simulink model "Group_11_Final_Project_model_ARO4090Rev4 (1)"  (R2023b)
settings: Solver=ode23tb  StartTime=0.0  StopTime=5676.8  FixedStep=0.002  RelTol=1e-3  EnableMultiTasking=on
undefined symbols (not defined in the file): IAU
libraries: simulink_extras x7, slpidlib x3, aerolibtransform2 x2, simulink x2
settings Model: ExtModeTrigDuration=10000  Creator=jtmil  LastModifiedBy=19095
settings SolverCC: AlgebraicLoopSolver=TrustRegion  PositivePriorityOrder=on
settings DataIOCC: ReturnWorkspaceOutputs=off
settings OptimizationCC: LifeSpan=inf
settings DebuggingCC: UnconnectedInputMsg=warning  UnconnectedOutputMsg=warning  UnconnectedLineMsg=warning  ArithmeticOperatorsInVariantConditions=warning
settings ModelReferenceCC: EnableRefExpFcnMdlSchedulingChecks=on
settings SFSimCC: SimUseLocalCustomCode=off  CustomCodeUndefinedFunction=UseInterfaceOnly
settings RTWCC: Description=QUARC Win64 Target  SystemTargetFile=quarc_win64.tlc  TemplateMakefile=quarc_default_tmf  RTWUseLocalCustomCode=off
settings CodeAppCC: StateflowObjectComments=on
settings STFCustomTargetCC: TargetPreCompLibLocation=C:\PROGRA~3\QUARC\lib\2016a\win64\release  ConcurrentExecutionCompliant=on  GRTInterface=on  SystemTargetFile=quarc_win64.tlc
settings GRTTargetCC: TargetPreCompLibLocation=C:\PROGRA~3\QUARC\lib\2016a\win64\release  ParMdlRefBuildCompliant=off  CompOptLevelCompliant=off  CombineOutputUpdateFcns=off  MatFileLogging=off  CPPClassGenCompliant=off  GRTInterface=on  UseToolchainInfoCompliant=off  ExtMode=on  ExtModeMexFile=quarc_comm
settings ConfigComp: CovMetricSettings=dswe

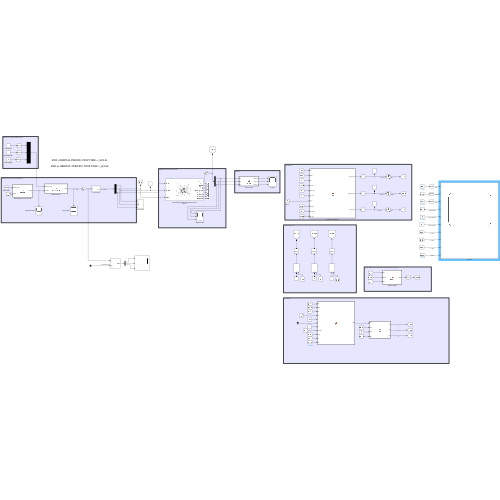
[thumbnail: Simulink's stored preview of the top-level diagram]
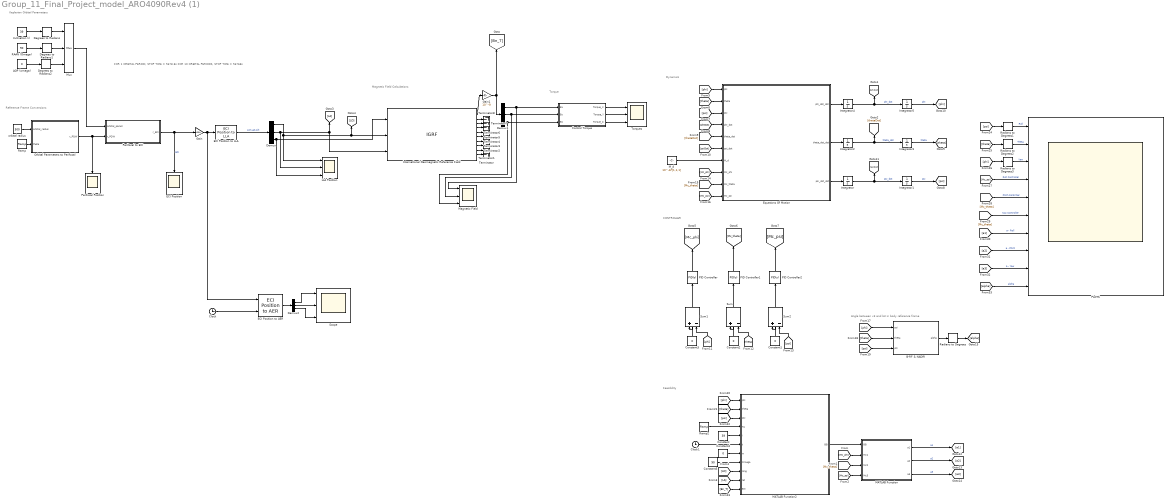
== system Group_11_Final_Project_model_ARO4090Rev4 (1) ==
  note: Feasibility
  note: Angle between v3 and b3 in body reference frame
  note: Dynamics
  note: CONTROLLER
  note: Torque
  note: Keplerian Orbital Parameters
  note: Magnetic Field Calculations
  note: Reference Frame Conversions
  note: FOR 1 ORBITAL PERIOD, STOP TIME = 5678.8s
      |
      | FOR 10 ORBITAL PERIODS, STOP TIME = 56768s
  AOP (omega) : Constant  Value=0
  B-RF & NADIR : MATLAB Function  TreatAsAtomicUnit=on
  Clock : Clock
  Clock1 : Clock
  Constant : Constant  Value=39
  Constant{1..4} (4 alike) : Constant  Value=0
  Constant5 : Constant  Value=90
  Control Torque : MATLAB Function  TreatAsAtomicUnit=on
  Degrees to Radians : simulink_extras/Transformations/Degrees to Radians
  Degrees to Radians1 : simulink_extras/Transformations/Degrees to Radians
  Degrees to Radians2 : simulink_extras/Transformations/Degrees to Radians
  Demux : Demux  Outputs=3
  Demux1 : Demux  Outputs=3
  Demux2 : Demux  Outputs=3
  ECI Position : Scope
  ECI Position to AER : aerolibtransform2/ECI Position to AER  red=IAU-2000/2006  year=2024  month=September  day=1  hour=0  min=0  sec=0  deltaT=Sec  errorflag=Error  extraparamflag=off  eunits=Metric (MKS)  earthmodel=WGS84  flat=1/298.257223563  eqradius=6378137  latlon0=[0 0]  psi0=0  href=0
      settings: AttributesFormatString=%<red>
  ECI Position to LLA : aerolibtransform2/ECI Position to LLA  red=IAU-2000/2006  year=2024  month=September  day=1  hour=0  min=0  sec=0  deltaT=None  errorflag=Error  extraparamflag=off  eunits=Metric (MKS)  earthmodel=WGS84  flat=1/298.257223563  eqradius=6378137
      settings: AttributesFormatString=%<red>
  Equations Of Motion : MATLAB Function  TreatAsAtomicUnit=on
  Gain : Gain  Gain=1000
  Gain1 : Gain  Gain=10^-9
  Inclination (i) : Constant  Value=39
  Integrator : Integrator
  Integrator1 : Integrator  InitialCondition=[.01]  WrapState=on
  Integrator2 : Integrator
  Integrator3 : Integrator  InitialCondition=[.01]  WrapState=on
  Integrator4 : Integrator
  Integrator5 : Integrator  InitialCondition=[.01]  WrapState=on
  International Geomagnetic Reference Field : IGRF  time_in=off  day=1  year=2024
      settings: AttributesFormatString=%<generation>
  LLA Position : Scope  NumInputPorts=3
  MATLAB Function : MATLAB Function  TreatAsAtomicUnit=on
  MATLAB Function2 : MATLAB Function  TreatAsAtomicUnit=on
  M_d : Constant  Value=10^-6*[1,1,1]
  Magnetic Field : Scope  NumInputPorts=3
  Mux : Mux  Inputs=3
  Orbital Parameters to Perifocal : MATLAB Function  TreatAsAtomicUnit=on
  PID Controller : slpidlib/PID Controller  Controller=PID  Form=Parallel  TimeDomain=Continuous-time  UseExternalTs=off  SampleTime=-1  IntegratorMethod=Forward Euler  FilterMethod=Forward Euler  ControllerParametersSource=internal  P=1.19311512336247e-06  I=1.08242545698123e-11  UseKiTs=off  D=0.0292205021506103  N=0.17771962118408  UseFilter=on  TunerSelectOption=Transfer Function Based (PID Tuner App)  InitialConditionSource=internal  InitialConditionForIntegrator=0  InitialConditionForFilter=0  DifferentiatorICPrevScaledInput=0  ExternalReset=none  TrackingMode=off  Kt=1  LimitOutput=off  SatLimitsSource=internal  UpperSaturationLimit=inf  LowerSaturationLimit=-inf  LinearizeAsGain=on  AntiWindupMode=none  Kb=1  LimitIntegrator=off  UpperIntegratorSaturationLimit=inf  LowerIntegratorSaturationLimit=-inf  POutMin=[]  POutMax=[]  IOutMin=[]  IOutMax=[]  DOutMin=[]  DOutMax=[]  NOutMin=[]  NOutMax=[]  SumOutMin=[]  SumOutMax=[]  SaturationOutMin=[]  SaturationOutMax=[]  PParamMin=[]  PParamMax=[]  IParamMin=[]  IParamMax=[]  DParamMin=[]  DParamMax=[]  NParamMin=[]  NParamMax=[]  KbParamMin=[]  KbParamMax=[]  KtParamMin=[]  KtParamMax=[]  KbOutMin=[]  KbOutMax=[]  KtOutMin=[]  KtOutMax=[]  IntegratorOutMin=[]  IntegratorOutMax=[]  FilterOutMin=[]  FilterOutMax=[]  SumI1OutMin=[]  SumI1OutMax=[]  SumI2OutMin=[]  SumI2OutMax=[]  SumI3OutMin=[]  SumI3OutMax=[]  SumI4OutMin=[]  SumI4OutMax=[]  SumDOutMin=[]  SumDOutMax=[]  DifferentiatorOutMin=[]  DifferentiatorOutMax=[]  FilterDiffOutCoefMin=[]  FilterDiffOutCoefMax=[]  ReciprocalOutMin=[]  ReciprocalOutMax=[]  SumDenOutMin=[]  SumDenOutMax=[]  SumNumOutMin=[]  SumNumOutMax=[]  DivideOutMin=[]  DivideOutMax=[]  UdiffTsProdOutMin=[]  UdiffTsProdOutMax=[]  NTsProdOutMin=[]  NTsProdOutMax=[]  UintegralTsProdOutMin=[]  UintegralTsProdOutMax=[]  UngainTsProdOutMin=[]  UngainTsProdOutMax=[]  ClampingZeroOutDataTypeStr=Inherit: Inherit via back propagation  ClampingZeroOutMin=[]  ClampingZeroOutMax=[]  FilterDenConstantOutDataTypeStr=Inherit: Inherit via back propagation  FilterDenConstantOutMin=[]  FilterDenConstantOutMax=[]  PCopyOutDataTypeStr=Inherit: Inherit via back propagation  PCopyOutMin=[]  PCopyOutMax=[]  NCopyOutDataTypeStr=Inherit: Inherit via back propagation  NCopyOutMin=[]  NCopyOutMax=[]  IntegratorContinuousStateAttributes=''  IntegratorStateMustResolveToSignalObject=off  IntegratorRTWStateStorageClass=Auto  FilterContinuousStateAttributes=''  FilterStateMustResolveToSignalObject=off  FilterRTWStateStorageClass=Auto  ParallelPVariant=InternalParameters  IdealPVariant=Disabled  IVariant=InternalParameters  DVariant=InternalParameters  IntegratorVariant=Continuous  SatVariant=Disabled  AWVariant=Passthrough  PCopyVariant=Disabled  TRVariant=Disabled  FdbkBlocksVariant=Forward  IdealPFdbkVariant=Disabled  SatFdbkVariant=Disabled  DerivativeFilterVariant=ContFilter  NVariant=InternalParameters  NCopyVariant=Disabled  FilterICVariant=InternalICsFilter  IntegratorICVariant=InternalICs  ExternalResetVariant=Disabled  TRSumVariant=Passthrough  SumFdbkVariant=Disabled  SumVariant=Sum_PID  TsampFilterVariant=InternalTs  TsampNgainVariant=Passthrough  TsampIntegralVariant=Disabled_SignalSpec  ExternalSaturationOutDataTypeStr=Inherit: Same as second input
  PID Controller1 : slpidlib/PID Controller  Controller=PID  Form=Parallel  TimeDomain=Continuous-time  UseExternalTs=off  SampleTime=-1  IntegratorMethod=Forward Euler  FilterMethod=Forward Euler  ControllerParametersSource=internal  P=0.00138798583925392  I=1.01724884485516e-06  UseKiTs=off  D=0.412850508107748  N=0.12618136735752  UseFilter=on  TunerSelectOption=Transfer Function Based (PID Tuner App)  InitialConditionSource=internal  InitialConditionForIntegrator=0  InitialConditionForFilter=0  DifferentiatorICPrevScaledInput=0  ExternalReset=none  TrackingMode=off  Kt=1  LimitOutput=off  SatLimitsSource=internal  UpperSaturationLimit=inf  LowerSaturationLimit=-inf  LinearizeAsGain=on  AntiWindupMode=none  Kb=1  LimitIntegrator=off  UpperIntegratorSaturationLimit=inf  LowerIntegratorSaturationLimit=-inf  POutMin=[]  POutMax=[]  IOutMin=[]  IOutMax=[]  DOutMin=[]  DOutMax=[]  NOutMin=[]  NOutMax=[]  SumOutMin=[]  SumOutMax=[]  SaturationOutMin=[]  SaturationOutMax=[]  PParamMin=[]  PParamMax=[]  IParamMin=[]  IParamMax=[]  DParamMin=[]  DParamMax=[]  NParamMin=[]  NParamMax=[]  KbParamMin=[]  KbParamMax=[]  KtParamMin=[]  KtParamMax=[]  KbOutMin=[]  KbOutMax=[]  KtOutMin=[]  KtOutMax=[]  IntegratorOutMin=[]  IntegratorOutMax=[]  FilterOutMin=[]  FilterOutMax=[]  SumI1OutMin=[]  SumI1OutMax=[]  SumI2OutMin=[]  SumI2OutMax=[]  SumI3OutMin=[]  SumI3OutMax=[]  SumI4OutMin=[]  SumI4OutMax=[]  SumDOutMin=[]  SumDOutMax=[]  DifferentiatorOutMin=[]  DifferentiatorOutMax=[]  FilterDiffOutCoefMin=[]  FilterDiffOutCoefMax=[]  ReciprocalOutMin=[]  ReciprocalOutMax=[]  SumDenOutMin=[]  SumDenOutMax=[]  SumNumOutMin=[]  SumNumOutMax=[]  DivideOutMin=[]  DivideOutMax=[]  UdiffTsProdOutMin=[]  UdiffTsProdOutMax=[]  NTsProdOutMin=[]  NTsProdOutMax=[]  UintegralTsProdOutMin=[]  UintegralTsProdOutMax=[]  UngainTsProdOutMin=[]  UngainTsProdOutMax=[]  ClampingZeroOutDataTypeStr=Inherit: Inherit via back propagation  ClampingZeroOutMin=[]  ClampingZeroOutMax=[]  FilterDenConstantOutDataTypeStr=Inherit: Inherit via back propagation  FilterDenConstantOutMin=[]  FilterDenConstantOutMax=[]  PCopyOutDataTypeStr=Inherit: Inherit via back propagation  PCopyOutMin=[]  PCopyOutMax=[]  NCopyOutDataTypeStr=Inherit: Inherit via back propagation  NCopyOutMin=[]  NCopyOutMax=[]  IntegratorContinuousStateAttributes=''  IntegratorStateMustResolveToSignalObject=off  IntegratorRTWStateStorageClass=Auto  FilterContinuousStateAttributes=''  FilterStateMustResolveToSignalObject=off  FilterRTWStateStorageClass=Auto  ParallelPVariant=InternalParameters  IdealPVariant=Disabled  IVariant=InternalParameters  DVariant=InternalParameters  IntegratorVariant=Continuous  SatVariant=Disabled  AWVariant=Passthrough  PCopyVariant=Disabled  TRVariant=Disabled  FdbkBlocksVariant=Forward  IdealPFdbkVariant=Disabled  SatFdbkVariant=Disabled  DerivativeFilterVariant=ContFilter  NVariant=InternalParameters  NCopyVariant=Disabled  FilterICVariant=InternalICsFilter  IntegratorICVariant=InternalICs  ExternalResetVariant=Disabled  TRSumVariant=Passthrough  SumFdbkVariant=Disabled  SumVariant=Sum_PID  TsampFilterVariant=InternalTs  TsampNgainVariant=Passthrough  TsampIntegralVariant=Disabled_SignalSpec  ExternalSaturationOutDataTypeStr=Inherit: Same as second input
  PID Controller2 : slpidlib/PID Controller  Controller=PID  Form=Parallel  TimeDomain=Continuous-time  UseExternalTs=off  SampleTime=-1  IntegratorMethod=Forward Euler  FilterMethod=Forward Euler  ControllerParametersSource=internal  P=1.79933480681122e-06  I=8.80958852713568e-11  UseKiTs=off  D=0.00363169506707376  N=0.00499000809163179  UseFilter=on  TunerSelectOption=Transfer Function Based (PID Tuner App)  InitialConditionSource=internal  InitialConditionForIntegrator=0  InitialConditionForFilter=0  DifferentiatorICPrevScaledInput=0  ExternalReset=none  TrackingMode=off  Kt=1  LimitOutput=off  SatLimitsSource=internal  UpperSaturationLimit=inf  LowerSaturationLimit=-inf  LinearizeAsGain=on  AntiWindupMode=none  Kb=1  LimitIntegrator=off  UpperIntegratorSaturationLimit=inf  LowerIntegratorSaturationLimit=-inf  POutMin=[]  POutMax=[]  IOutMin=[]  IOutMax=[]  DOutMin=[]  DOutMax=[]  NOutMin=[]  NOutMax=[]  SumOutMin=[]  SumOutMax=[]  SaturationOutMin=[]  SaturationOutMax=[]  PParamMin=[]  PParamMax=[]  IParamMin=[]  IParamMax=[]  DParamMin=[]  DParamMax=[]  NParamMin=[]  NParamMax=[]  KbParamMin=[]  KbParamMax=[]  KtParamMin=[]  KtParamMax=[]  KbOutMin=[]  KbOutMax=[]  KtOutMin=[]  KtOutMax=[]  IntegratorOutMin=[]  IntegratorOutMax=[]  FilterOutMin=[]  FilterOutMax=[]  SumI1OutMin=[]  SumI1OutMax=[]  SumI2OutMin=[]  SumI2OutMax=[]  SumI3OutMin=[]  SumI3OutMax=[]  SumI4OutMin=[]  SumI4OutMax=[]  SumDOutMin=[]  SumDOutMax=[]  DifferentiatorOutMin=[]  DifferentiatorOutMax=[]  FilterDiffOutCoefMin=[]  FilterDiffOutCoefMax=[]  ReciprocalOutMin=[]  ReciprocalOutMax=[]  SumDenOutMin=[]  SumDenOutMax=[]  SumNumOutMin=[]  SumNumOutMax=[]  DivideOutMin=[]  DivideOutMax=[]  UdiffTsProdOutMin=[]  UdiffTsProdOutMax=[]  NTsProdOutMin=[]  NTsProdOutMax=[]  UintegralTsProdOutMin=[]  UintegralTsProdOutMax=[]  UngainTsProdOutMin=[]  UngainTsProdOutMax=[]  ClampingZeroOutDataTypeStr=Inherit: Inherit via back propagation  ClampingZeroOutMin=[]  ClampingZeroOutMax=[]  FilterDenConstantOutDataTypeStr=Inherit: Inherit via back propagation  FilterDenConstantOutMin=[]  FilterDenConstantOutMax=[]  PCopyOutDataTypeStr=Inherit: Inherit via back propagation  PCopyOutMin=[]  PCopyOutMax=[]  NCopyOutDataTypeStr=Inherit: Inherit via back propagation  NCopyOutMin=[]  NCopyOutMax=[]  IntegratorContinuousStateAttributes=''  IntegratorStateMustResolveToSignalObject=off  IntegratorRTWStateStorageClass=Auto  FilterContinuousStateAttributes=''  FilterStateMustResolveToSignalObject=off  FilterRTWStateStorageClass=Auto  ParallelPVariant=InternalParameters  IdealPVariant=Disabled  IVariant=InternalParameters  DVariant=InternalParameters  IntegratorVariant=Continuous  SatVariant=Disabled  AWVariant=Passthrough  PCopyVariant=Disabled  TRVariant=Disabled  FdbkBlocksVariant=Forward  IdealPFdbkVariant=Disabled  SatFdbkVariant=Disabled  DerivativeFilterVariant=ContFilter  NVariant=InternalParameters  NCopyVariant=Disabled  FilterICVariant=InternalICsFilter  IntegratorICVariant=InternalICs  ExternalResetVariant=Disabled  TRSumVariant=Passthrough  SumFdbkVariant=Disabled  SumVariant=Sum_PID  TsampFilterVariant=InternalTs  TsampNgainVariant=Passthrough  TsampIntegralVariant=Disabled_SignalSpec  ExternalSaturationOutDataTypeStr=Inherit: Same as second input
  PLOTS : Scope  NumInputPorts=10
  Perifocal Position : Scope
  Perifocal to ECI : MATLAB Function  TreatAsAtomicUnit=on
  RAAN (Omega) : Constant  Value=90
  Radians to Degrees{,1..3} (4 alike) : simulink_extras/Transformations/Radians to Degrees
  Ramp : simulink/Sources/Ramp  slope=360/5676.8  start=0  InitialOutput=0
  Ramp2 : simulink/Sources/Ramp  slope=360/5676.8  start=0  InitialOutput=0
  Scope : Scope  NumInputPorts=3
  Sum : Sum  Inputs=|+-
  Sum1 : Sum  Inputs=|+-
  Sum2 : Sum  Inputs=|+-
  Terminator{,1..8} (9 alike) : Terminator
  Torques : Scope  NumInputPorts=3
  orbital radius : Constant  Value=500
  wires:
  Demux1/2 -> Magnetic Field/2, Control Torque/2(By)
  Control Torque/1(Torque_X) -> Torques/1
  International Geomagnetic Reference Field/5 -> Terminator5/1
  International Geomagnetic Reference Field/4 -> Terminator6/1
  Degrees to Radians2/1 -> Mux/3
  Gain/1 -> ECI Position to AER/1, ECI Position to LLA/1
  Control Torque/3(Torque_Z) -> Torques/3
  Degrees to Radians1/1 -> Mux/2
  International Geomagnetic Reference Field/10 -> Terminator/1
  International Geomagnetic Reference Field/3 -> Terminator7/1
  Demux1/3 -> Control Torque/3(Bz), Magnetic Field/3
  International Geomagnetic Reference Field/9 -> Terminator1/1
  Demux/2 -> International Geomagnetic Reference Field/3, [LA], LLA Position/2
  Demux/1 -> [LO], International Geomagnetic Reference Field/2, LLA Position/1
  Demux1/1 -> Magnetic Field/1, Control Torque/1(Bx)
  Mux/1 -> Perifocal to ECI/1(orbital_param)
  Control Torque/2(Torque_Y) -> Torques/2
  Perifocal to ECI/1(r_ECI) -> Gain/1, ECI Position/1  "ECI"
  Degrees to Radians/1 -> Mux/1
  Ramp/1 -> Orbital Parameters to Perifocal/2(theta)
  International Geomagnetic Reference Field/7 -> Terminator3/1
  ECI Position to LLA/1 -> Demux/1  "Lon,Lat,Alt"
  International Geomagnetic Reference Field/6 -> Terminator4/1
  International Geomagnetic Reference Field/8 -> Terminator2/1
  Demux/3 -> International Geomagnetic Reference Field/1, LLA Position/3
  International Geomagnetic Reference Field/2 -> Terminator8/1
  Inclination (i)/1 -> Degrees to Radians/1
  Orbital Parameters to Perifocal/1(r_PQW) -> Perifocal to ECI/2(r_PQW), Perifocal Position/1
  RAAN (Omega)/1 -> Degrees to Radians1/1
  orbital radius/1 -> Orbital Parameters to Perifocal/1(orbital_radius)
  AOP (omega)/1 -> Degrees to Radians2/1
  Integrator/1 -> [psiDot], Integrator1/1  "psi_dot"
  Integrator2/1 -> [thetaDot], Integrator3/1  "theta_dot"
  Integrator4/1 -> Integrator5/1, [phiDot]  "phi_dot"
  Equations Of Motion/3(psi_dot_dot) -> Integrator/1
  Equations Of Motion/2(theta_dot_dot) -> Integrator2/1
  Equations Of Motion/1(phi_dot_dot) -> Integrator4/1
  M_d/1 -> Equations Of Motion/7(M_d)
  Clock/1 -> ECI Position to AER/2
  ECI Position to AER/1 -> Demux2/1
  Demux2/1 -> Scope/1
  Demux2/2 -> Scope/2
  Demux2/3 -> Scope/3
  Sum2/1 -> PID Controller2/1
  Sum/1 -> PID Controller1/1
  Constant1/1 -> Sum2/1
  Constant2/1 -> Sum/1
  Constant3/1 -> Sum1/1
  B-RF & NADIR/1(alpha) -> Radians to Degrees/1
  Radians to Degrees/1 -> [alpha]
  Ramp2/1 -> MATLAB Function2/4(TA)
  Constant/1 -> MATLAB Function2/5(i)
  Constant4/1 -> MATLAB Function2/7(w)
  Constant5/1 -> MATLAB Function2/8(Omega)
  [LA] -> MATLAB Function2/10(lat)
  [LO] -> MATLAB Function2/9(long)
  MATLAB Function2/1(BB) -> MATLAB Function/1(BB)
  [Mc_phi] -> MATLAB Function/2(Mc1)
  [Mc_theta] -> MATLAB Function/3(Mc2)
  [Mc_psi] -> MATLAB Function/4(Mc3)
  MATLAB Function/1(a1) -> [a1]  "a1"
  MATLAB Function/2(a2) -> [a2]  "a2"
  MATLAB Function/3(a3) -> [a3]  "a3"
  Clock1/1 -> MATLAB Function2/6(t)
  Sum1/1 -> PID Controller/1
  Integrator5/1 -> [phi]  "phi"
  Integrator3/1 -> [theta]  "theta"
  Integrator1/1 -> [psi]  "psi"
  [phi] -> Equations Of Motion/1(phi)
  [theta] -> Equations Of Motion/2(theta)
  [psi] -> Equations Of Motion/3(psi)
  [phiDot] -> Equations Of Motion/4(phi_dot)
  [thetaDot] -> Equations Of Motion/5(theta_dot)
  [psiDot] -> Equations Of Motion/6(psi_dot)
  PID Controller2/1 -> [Mc_psi]
  PID Controller1/1 -> [Mc_theta]
  PID Controller/1 -> [Mc_phi]
  [phi] -> Sum1/2
  [theta] -> Sum/2
  [psi] -> Sum2/2
  [Mc_phi] -> Equations Of Motion/8(Mc_phi)
  [Mc_theta] -> Equations Of Motion/9(Mc_theta)
  [Mc_psi] -> Equations Of Motion/10(Mc_psi)
  [theta] -> B-RF & NADIR/2(theta)
  [phi] -> B-RF & NADIR/1(psi)
  [psi] -> B-RF & NADIR/3(phi)
  [phi] -> MATLAB Function2/1(phi)
  [psi] -> MATLAB Function2/3(psi)
  [theta] -> MATLAB Function2/2(theta)
  International Geomagnetic Reference Field/1 -> Gain1/1
  Gain1/1 -> Demux1/1, [Bn_T]
  [Bn_T] -> MATLAB Function2/11(BN)
  [psi] -> Radians to Degrees1/1
  [theta] -> Radians to Degrees2/1
  [phi] -> Radians to Degrees3/1
  [Mc_psi] -> PLOTS/4  "Roll Controller"
  [Mc_theta] -> PLOTS/5  "Pitch Contriller"
  [Mc_theta] -> PLOTS/6  "Yaw Controller"
  [a1] -> PLOTS/7  "a - Roll"
  [a2] -> PLOTS/8  "a - Pitch"
  [a3] -> PLOTS/9  "a - Yaw"
  Radians to Degrees1/1 -> PLOTS/1  "Roll"
  Radians to Degrees2/1 -> PLOTS/2  "Theta"
  Radians to Degrees3/1 -> PLOTS/3  "Yaw"
  [alpha] -> PLOTS/10  "alpha"

== matlab function Group_11_Final_Project_model_ARO4090Rev4 (1)/Perifocal to ECI ==
  data: orbital_param input; r_ECI output; r_PQW input
function r_ECI = Perifocal2ECI(orbital_param , r_PQW)

i = orbital_param(1);
Omega = orbital_param(2);
omega = orbital_param(3);

R3_Omega = [cos(Omega), -sin(Omega), 0; sin(Omega), cos(Omega), 0; 0, 0, 1];
R1_i = [1, 0, 0; 0, cos(i), -sin(i); 0, sin(i), cos(i)];
R3_omega = [cos(omega), -sin(omega), 0; sin(omega), cos(omega), 0; 0, 0, 1];

R_PQW_to_ECI = R3_Omega * R1_i * R3_omega;


% Transform to ECI coordinates
r_ECI = R_PQW_to_ECI * r_PQW;

== matlab function Group_11_Final_Project_model_ARO4090Rev4 (1)/Orbital Parameters to Perifocal ==
  data: orbital_radius input; r_PQW output; theta input
function r_PQW = Perifocal(orbital_radius,theta)


Earth_Radius = 6378;

Orbital_Radius = orbital_radius + Earth_Radius;


r_PQW = [Orbital_Radius * cosd(theta); Orbital_Radius * sind(theta); zeros(1, length(theta))];


end

== matlab function Group_11_Final_Project_model_ARO4090Rev4 (1)/Control Torque ==
  data: Bx input; Torque_X output; By input; Bz input; Torque_Y output; Torque_Z output
function [Torque_X,Torque_Y,Torque_Z] = Torque(Bx,By,Bz)

m_IB = [0.2 ; 0 ; 0] ;      % magnetorque - x_axis (Am^2)
m_YB = [0 ; 0.2 ; 0] ;      % magnetorque - y_axis (Am^2)
m_ZB = [0 ; 0 ; 0.1] ;      % magnetorque - z_axis (Am^2)

m = norm([m_IB , m_YB , m_ZB ]);

Torque_X = norm(m_IB)*Bx*sind(45);
Torque_Y = norm(m_YB)*By*sind(45);
Torque_Z = norm(m_ZB)*Bz*sind(45);


end

== matlab function Group_11_Final_Project_model_ARO4090Rev4 (1)/Equations Of Motion ==
  data: phi input; theta input; psi input; phi_dot input; theta_dot input; psi_dot input; M_d input; phi_dot_dot output; theta_dot_dot output; psi_dot_dot output; Mc_phi input; Mc_theta input; Mc_psi input
function [phi_dot_dot , theta_dot_dot , psi_dot_dot] = fcn(phi,theta,psi,phi_dot,theta_dot,psi_dot,M_d, Mc_phi, Mc_theta, Mc_psi)

% w_0 = sqrt(mu/(R_c)^3 Lecture 20/21

Ixx = 36.5;
Iyy = 36.5;
Izz = 9.21;

w_0 = sqrt(398600 / 6878^3);     % [ rad / s ]

phi_dot_dot =(1/Ixx)* ((Ixx-Iyy+Izz)*w_0*psi_dot - (Iyy-Izz)*4*phi*w_0^2 + M_d(1) + Mc_phi);        % Roll Eq.

theta_dot_dot = (1/Iyy)*(  M_d(2) - (Ixx-Izz)*3*theta*w_0^2 + Mc_theta);                             % Pitch Eq.

psi_dot_dot = (1/Izz)*( M_d(3) - (Ixx-Iyy+Izz)*phi_dot*w_0 - (Iyy-Izz)*phi*w_0^2 + Mc_psi);          % Yaw Eq.

end

== matlab function Group_11_Final_Project_model_ARO4090Rev4 (1)/B-RF & NADIR ==
  data: psi input; alpha output size=1; theta input; phi input
function alpha = vDOTb(psi, theta, phi)

    Rbv = [cos(theta) * cos(psi), cos(theta) * sin(psi), -sin(theta);
            sin(phi)*sin(theta)*cos(psi) - cos(phi)*sin(psi), sin(phi)*sin(theta)*sin(psi) + cos(phi)*cos(psi), sin(phi)*cos(theta);
            cos(phi)*sin(theta)*cos(psi) + sin(phi)*sin(psi), cos(phi)*sin(theta)*sin(psi) - sin(phi)*cos(psi), cos(phi)*cos(theta)];

    v3_v = [0;0;1];
    v3_b = Rbv * v3_v;
    
    dotproduct = dot(v3_v, v3_b);
        
    alpha = acos(dotproduct);


end

== matlab function Group_11_Final_Project_model_ARO4090Rev4 (1)/MATLAB Function ==
  data: BB input; a1 output; Mc1 input; Mc2 input; Mc3 input; a2 output; a3 output
function [a1 , a2 , a3] = fcn(BB, Mc1 , Mc2 , Mc3)

% a^T = diag

mx = [0.2 , 0 , 0];
my = [0 , 0.2 , 0];
mz = [0 , 0 , 0.1];

m_matrix = [1/norm(mx) , 0 , 0;
                0 , 1/norm(my), 0;
                0 , 0 , 1/norm(mz)];
Bnormalized = BB*(1/norm(BB)^2)

Mc = [Mc1 ; Mc2 ; Mc3];

a = m_matrix*cross(Mc,Bnormalized);

a1 = a(1);
a2 = a(2);
a3 = a(3);







end

== matlab function Group_11_Final_Project_model_ARO4090Rev4 (1)/MATLAB Function2 ==
  data: phi input; theta input; psi input; TA input; i input; t input; w input; Omega input; long input; lat input; BN input; BB output
function BB  = fcn(phi, theta, psi, TA, i,t, w, Omega, long, lat,BN)

    

    R1rvp = [1, 0, 0; 0, cos(phi), sin(phi); 0, -sin(phi), cos(phi)];
    R2rvp = [cos(theta), 0, -sin(theta); 0, 1, 0; sin(theta), 0, cos(theta)];
    R3rvp = [cos(psi), sin(psi), 0; -sin(psi), cos(psi), 0; 0, 0, 1];

    R2ta = [cosd(TA), 0, -sind(TA); 0, 1, 0; sind(TA), 0, cosd(TA)];
    R3ta = [cosd(90), sind(90), 0; -sind(90), cosd(90), 0; 0, 0, 1];
    R2ta2 = [cosd(-90), 0, -sind(-90); 0, 1, 0; sind(-90), 0, cosd(-90)];

    R3rpi = [cosd(w), sind(w), 0; -sind(w), cosd(w), 0; 0, 0, 1];
    R1rpi = [1, 0, 0; 0, cosd(i), sind(i); 0, -sind(i), cosd(i)];
    R3rpi2 = [cosd(Omega), sind(Omega), 0; -sind(Omega), cosd(Omega), 0; 0, 0, 1];

    R3long = [cosd(long), sind(long), 0; -sind(long), cosd(long), 0; 0, 0, 1];
    R2lat = [cosd(lat + 90), 0, -sind(lat + 90); 0, 1, 0; sind(lat + 90), 0, cosd(lat + 90)];
 

% Find Theta_g0 - [Found from relations in curtis J0 -> T0 - > thetaG0 ]
% y = 2024;
% m = 9;
% d = 1
% 
%     J0 = 367*y - fix(7/4*(y+fix((m+9)/12))) + fix(275*m/9) + d + 1721013.5;
% 
%     T0 = (J0-2451545)/36525;
% 
%     thetaG0 = mod(100.4606184 + 36000.77004*T0 + 3.87933E-4*T0^2 - 2.583E-8*T0^3,360);

thetaG0 = 340.650585203182;

theta_g_t = thetaG0 + (360/86164)*t;

 R3g = [cosd(-theta_g_t), sind(-theta_g_t), 0; -sin(-theta_g_t), cos(-theta_g_t), 0; 0, 0, 1];

    % Rotation Matrices

    Rbv = R1rvp * R2rvp * R3rvp;
    Rvp = R2ta * R3ta * R2ta2;
    Rpi = R3rpi * R1rpi * R3rpi2;
    Rif = R3g;
    Rfn = R3long * R2lat;
    Rbn = Rbv * Rvp * Rpi * Rif * Rfn;
    
BB = Rbn*BN;

end
